simulink model "qtest1"  (Simulink 7.0)
settings: Solver=FixedStepDiscrete  StartTime=0.0  StopTime=1.0  FixedStep=1.0  RelTol=1e-3
values from neighbouring files (symbols this model uses):
  sim_q = q    [unit_test.m]
  sim_v = v    [unit_test.m]
libraries: qlib x10
settings Model: Creator=stpierre  LastModifiedBy=stpierre  ExtModeAutoUpdateStatusClock=off

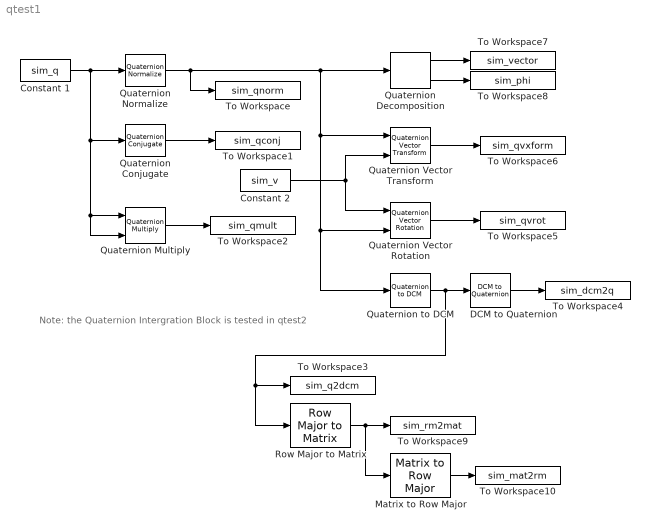
== system qtest1 ==
  note: Note: the Quaternion Intergration
      | Block is tested in qtest2
  Constant 1 : Constant  Value=sim_q
  Constant 2 : Constant  Value=sim_v
  DCM to Quaternion : qlib/DCM to Quaternion  SystemSampleTime=-1
  Matrix to Row Major : qlib/Matrix to Row Major  SystemSampleTime=-1
  Quaternion Conjugate : qlib/Quaternion Conjugate  SystemSampleTime=-1
  Quaternion Decomposition : qlib/Quaternion Decomposition  SystemSampleTime=-1
  Quaternion Multiply : qlib/Quaternion Multiply  SystemSampleTime=-1
  Quaternion Normalize : qlib/Quaternion Normalize  SystemSampleTime=-1
  Quaternion Vector Rotation : qlib/Quaternion Vector Rotation  SystemSampleTime=-1
  Quaternion Vector Transform : qlib/Quaternion Vector Transform  SystemSampleTime=-1
  Quaternion to DCM : qlib/Quaternion to DCM  SystemSampleTime=-1
  Row Major to Matrix : qlib/Row Major to Matrix  SystemSampleTime=-1  rows=3  columns=3
  To Workspace : ToWorkspace  VariableName=sim_qnorm  SampleTime=-1  SaveFormat=Array
      settings: MaxDataPoints=1
  To Workspace1 : ToWorkspace  VariableName=sim_qconj  SampleTime=-1  SaveFormat=Array
      settings: MaxDataPoints=1
  To Workspace10 : ToWorkspace  VariableName=sim_mat2rm  SampleTime=-1  SaveFormat=Array
      settings: MaxDataPoints=1
  To Workspace2 : ToWorkspace  VariableName=sim_qmult  SampleTime=-1  SaveFormat=Array
      settings: MaxDataPoints=1
  To Workspace3 : ToWorkspace  VariableName=sim_q2dcm  SampleTime=-1  SaveFormat=Array
      settings: MaxDataPoints=1
  To Workspace4 : ToWorkspace  VariableName=sim_dcm2q  SampleTime=-1  SaveFormat=Array
      settings: MaxDataPoints=1
  To Workspace5 : ToWorkspace  VariableName=sim_qvrot  SampleTime=-1  SaveFormat=Array
      settings: MaxDataPoints=1
  To Workspace6 : ToWorkspace  VariableName=sim_qvxform  SampleTime=-1  SaveFormat=Array
      settings: MaxDataPoints=1
  To Workspace7 : ToWorkspace  VariableName=sim_vector  SampleTime=-1  SaveFormat=Array
      settings: MaxDataPoints=1
  To Workspace8 : ToWorkspace  VariableName=sim_phi  SampleTime=-1  SaveFormat=Array
      settings: MaxDataPoints=1
  To Workspace9 : ToWorkspace  VariableName=sim_rm2mat  SampleTime=-1  SaveFormat=Array
      settings: MaxDataPoints=1
  wires:
  Constant 1/1 -> Quaternion Multiply/2, Quaternion Multiply/1, Quaternion Conjugate/1, Quaternion Normalize/1
  Quaternion Normalize/1 -> Quaternion to DCM/1, Quaternion Vector Rotation/2, Quaternion Vector Transform/1, Quaternion Decomposition/1, To Workspace/1
  Quaternion Conjugate/1 -> To Workspace1/1
  Quaternion Multiply/1 -> To Workspace2/1
  Quaternion to DCM/1 -> DCM to Quaternion/1, To Workspace3/1, Row Major to Matrix/1
  DCM to Quaternion/1 -> To Workspace4/1
  Quaternion Vector Rotation/1 -> To Workspace5/1
  Quaternion Vector Transform/1 -> To Workspace6/1
  Quaternion Decomposition/1 -> To Workspace7/1
  Quaternion Decomposition/2 -> To Workspace8/1
  Constant 2/1 -> Quaternion Vector Rotation/1, Quaternion Vector Transform/2
  Row Major to Matrix/1 -> To Workspace9/1, Matrix to Row Major/1
  Matrix to Row Major/1 -> To Workspace10/1
